simulink model "simulink_validacao"  (R2016a)
settings: Solver=VariableStepAuto  StartTime=0.0  StopTime=10.0  RelTol=1e-3
values from neighbouring files (symbols this model uses):
  f_mol_ar = [0.79 0.21 0.0 0 0 0 0 0]    [codigo_validacao.m]
  f_mol_gas = [0.76 0 0 0 0.11 0.13 0 0]    [codigo_validacao.m]
  m_c = 0.3    [codigo_validacao.m]
  m_f = 0.01    [codigo_validacao.m]
  N = 0.82    [codigo_validacao.m]
  Pc_i = 368000    [codigo_validacao.m]
  Ph_i = 105000    [codigo_validacao.m]
  Tc_i = 358.15    [codigo_validacao.m]
  Th_i = 584.817    [codigo_validacao.m]
(part 2 of 4)

== system simulink_validacao/Recuperdor de calor CWPS/Troca de Calor/Coef. Convectivo ==
  k_ar [W/m.K] : Inport
  k_gas [W/m.K] : Inport  Port=2
  nu_ar : Inport  Port=3
  nu_gas : Inport  Port=4
  dh_ar [m] : Inport  Port=5
  dh_gas [m] : Inport  Port=6
  Coeficiente Convectivo fluido frio : Fcn  Expr=u(1)*u(2)*(1/u(3))
  Coeficiente Convectivo fluido quente : Fcn  Expr=u(1)*u(2)*(1/u(3))
  Mux1 : Mux  Inputs=3
  Mux2 : Mux  Inputs=3
  coef-h_c [W/(m2.K)] : Outport
  coef-h_h [W/(m2.K)] : Outport  Port=2
  wires:
  nu_ar/1 -> Mux1/1
  nu_gas/1 -> Mux2/1
  k_ar [W/m.K]/1 -> Mux1/2
  k_gas [W/m.K]/1 -> Mux2/2
  Mux1/1 -> Coeficiente Convectivo fluido frio/1
  Coeficiente Convectivo fluido frio/1 -> coef-h_c [W/(m2.K)]/1
  dh_gas [m]/1 -> Mux2/3
  dh_ar [m]/1 -> Mux1/3
  Coeficiente Convectivo fluido quente/1 -> coef-h_h [W/(m2.K)]/1
  Mux2/1 -> Coeficiente Convectivo fluido quente/1

== system simulink_validacao/Recuperdor de calor CWPS/Troca de Calor/Coef. global ==
  coef-h_c [W/(m2.K)] : Inport
  coef-h_h [W/(m2.K)] : Inport  Port=2
  Calc. Coef. global : Fcn  Expr=(1/(u(1)*u(2)))+(1/(u(3)*u(4)))
  Mux1 : Mux
  cg [K/W] : Outport
  wires:
  coef-h_c [W/(m2.K)]/1 -> Mux1/1
  [Aht_h] -> Mux1/4
  coef-h_h [W/(m2.K)]/1 -> Mux1/3
  Calc. Coef. global/1 -> cg [K/W]/1
  Mux1/1 -> Calc. Coef. global/1
  [Aht_c] -> Mux1/2

== system simulink_validacao/Recuperdor de calor CWPS/Troca de Calor/Condutividade ==
  t_c_i [K] : Inport
  t_c_o [K] : Inport  Port=2
  t_h_i [K] : Inport  Port=3
  t_h_o [K] : Inport  Port=4
  Mux : Mux  Inputs=2
  Mux1 : Mux  Inputs=2
  T media fluido frio : Fcn  Expr=(u(1)+u(2))/2
  T media fluido quente : Fcn  Expr=(u(1)+u(2))/2
  cond_c_ch : MATLAB Function  TreatAsAtomicUnit=on
  cond_c_ch1 : MATLAB Function  TreatAsAtomicUnit=on
  k_c_ch [W/m.K] : Outport
  k_h_ch [W/m.K] : Outport  Port=2
  wires:
  Mux/1 -> T media fluido frio/1
  t_c_i [K]/1 -> Mux/1
  t_c_o [K]/1 -> Mux/2
  T media fluido frio/1 -> cond_c_ch/1(t)
  cond_c_ch/1(y) -> k_c_ch [W/m.K]/1
  Mux1/1 -> T media fluido quente/1
  t_h_i [K]/1 -> Mux1/1
  t_h_o [K]/1 -> Mux1/2
  T media fluido quente/1 -> cond_c_ch1/1(t)
  cond_c_ch1/1(y) -> k_h_ch [W/m.K]/1
  [f_mol_c] -> cond_c_ch/2(frac_mol)
  [f_mol_h] -> cond_c_ch1/2(frac_mol)

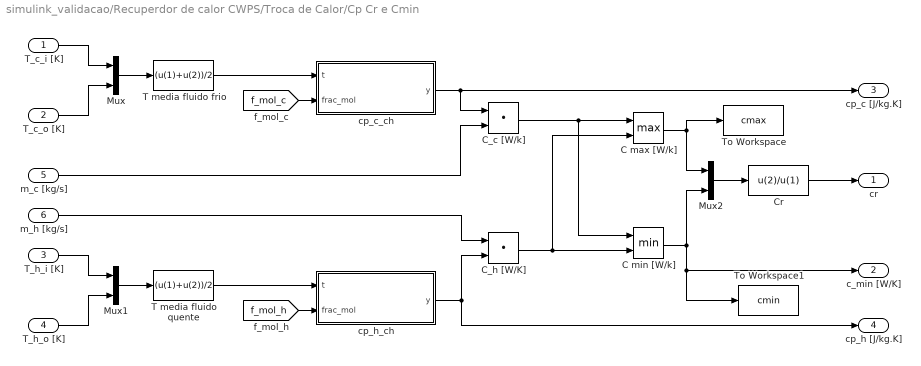
== system simulink_validacao/Recuperdor de calor CWPS/Troca de Calor/Cp Cr e Cmin ==
  T_c_i [K] : Inport
  T_c_o [K] : Inport  Port=2
  T_h_i [K] : Inport  Port=3
  T_h_o [K] : Inport  Port=4
  m_c [kg/s] : Inport  Port=5
  m_h [kg/s] : Inport  Port=6
  C max [W/k] : MinMax  Function=max  Inputs=2
  C min [W/k] : MinMax  Inputs=2
  C_c [W/k] : DotProduct  InputSameDT=on  OutDataTypeStr=Inherit: Inherit via internal rule
  C_h [W/K] : DotProduct  InputSameDT=on  OutDataTypeStr=Inherit: Inherit via internal rule
  Cr : Fcn  Expr=u(2)/u(1)
  Mux : Mux  Inputs=2
  Mux1 : Mux  Inputs=2
  Mux2 : Mux  Inputs=2
  T media fluido frio : Fcn  Expr=(u(1)+u(2))/2
  T media fluido quente : Fcn  Expr=(u(1)+u(2))/2
  To Workspace : ToWorkspace  VariableName=cmax  SampleTime=-1
      settings: Save2DSignal=2-D array (concatenate along first dimension)
  To Workspace1 : ToWorkspace  VariableName=cmin  SampleTime=-1
      settings: Save2DSignal=2-D array (concatenate along first dimension)
  cp_c_ch : MATLAB Function  TreatAsAtomicUnit=on
  cp_h_ch : MATLAB Function  TreatAsAtomicUnit=on
  cr : Outport
  c_min [W/K] : Outport  Port=2
  cp_c [J/kg.K] : Outport  Port=3
  cp_h [J/kg.K] : Outport  Port=4
  wires:
  Mux/1 -> T media fluido frio/1
  T_c_i [K]/1 -> Mux/1
  m_h [kg/s]/1 -> C_h [W/K]/1
  T media fluido quente/1 -> cp_h_ch/1(t)
  T_h_i [K]/1 -> Mux1/1
  C max [W/k]/1 -> Mux2/1, To Workspace/1
  cp_h_ch/1(y) -> C_h [W/K]/2, cp_h [J/kg.K]/1
  m_c [kg/s]/1 -> C_c [W/k]/2
  C_c [W/k]/1 -> C min [W/k]/1, C max [W/k]/1
  Cr/1 -> cr/1
  T_c_o [K]/1 -> Mux/2
  cp_c_ch/1(y) -> cp_c [J/kg.K]/1, C_c [W/k]/1
  T_h_o [K]/1 -> Mux1/2
  Mux2/1 -> Cr/1
  C_h [W/K]/1 -> C min [W/k]/2, C max [W/k]/2
  T media fluido frio/1 -> cp_c_ch/1(t)
  Mux1/1 -> T media fluido quente/1
  C min [W/k]/1 -> To Workspace1/1, c_min [W/K]/1, Mux2/2
  [f_mol_c] -> cp_c_ch/2(frac_mol)
  [f_mol_h] -> cp_h_ch/2(frac_mol)

== system simulink_validacao/Recuperdor de calor CWPS/Troca de Calor/Efetividade ==
  cr : Inport
  nut : Inport  Port=2
  Calc. Efetividade : Fcn  Expr=(1-exp(-u(2)*(1-u(1))))/(1-u(1)*exp(-u(2)*(1-u(1))))
  Mux1 : Mux  Inputs=2
  efetividade : ToWorkspace  VariableName=efetiv  SampleTime=-1
      settings: Save2DSignal=2-D array (concatenate along first dimension)
  epsilon : Outport
  wires:
  nut/1 -> Mux1/2
  cr/1 -> Mux1/1
  Calc. Efetividade/1 -> efetividade/1, epsilon/1
  Mux1/1 -> Calc. Efetividade/1

== system simulink_validacao/Recuperdor de calor CWPS/Troca de Calor/NUT ==
  c_min [W/K] : Inport
  cg [K/W] : Inport  Port=2
  Calc. NUT : Fcn  Expr=1/(u(1)*u(2))
  Mux1 : Mux  Inputs=2
  nut : Outport
  wires:
  cg [K/W]/1 -> Mux1/2
  c_min [W/K]/1 -> Mux1/1
  Calc. NUT/1 -> nut/1
  Mux1/1 -> Calc. NUT/1

== system simulink_validacao/Recuperdor de calor CWPS/Troca de Calor/Nusselt ==
  pr_ar : Inport
  pr_gas : Inport  Port=2
  re_ar : Inport  Port=3
  re_gas : Inport  Port=4
  Calc. Nusselt ar : Fcn  Expr=0.0031*(u(1)^1.18)*(u(2)^0.4)*((2*u(3)/u(4))^0.19)
  Calc. Nusselt gas : Fcn  Expr=0.0031*(u(1)^1.18)*(u(2)^0.4)*((2*u(3)/u(4))^0.19)
  Mux1 : Mux
  Mux2 : Mux
  nu_ar : Outport
  nu_gas : Outport  Port=2
  wires:
  pr_ar/1 -> Mux1/2
  Mux2/1 -> Calc. Nusselt gas/1
  Calc. Nusselt gas/1 -> nu_gas/1
  re_ar/1 -> Mux1/1
  re_gas/1 -> Mux2/1
  [W_c] -> Mux1/4
  [h] -> Mux2/3, Mux1/3
  Calc. Nusselt ar/1 -> nu_ar/1
  Mux1/1 -> Calc. Nusselt ar/1
  [W_h] -> Mux2/4
  pr_gas/1 -> Mux2/2

== system simulink_validacao/Recuperdor de calor CWPS/Troca de Calor/Prandlt ==
  cp_ar [J/kg.K] : Inport
  cp_gas [J/kg.K] : Inport  Port=2
  mu_ar [kg/m.s] : Inport  Port=3
  mu_gas [kg/m.s] : Inport  Port=4
  k_ar_ch [W/m.K] : Inport  Port=5
  k_gas_ch  [W/m.K] : Inport  Port=6
  Mux : Mux  Inputs=3
  Mux1 : Mux  Inputs=3
  Prandlt fluido frio : Fcn  Expr=(u(1)*u(2))/(u(3))
  Prandlt fluido quente : Fcn  Expr=(u(1)*u(2))/(u(3))
  pr_c : Outport
  pr_h : Outport  Port=2
  wires:
  Mux1/1 -> Prandlt fluido quente/1
  Prandlt fluido quente/1 -> pr_h/1
  k_gas_ch  [W/m.K]/1 -> Mux1/3
  cp_gas [J/kg.K]/1 -> Mux1/1
  mu_ar [kg/m.s]/1 -> Mux/2
  Mux/1 -> Prandlt fluido frio/1
  Prandlt fluido frio/1 -> pr_c/1
  mu_gas [kg/m.s]/1 -> Mux1/2
  cp_ar [J/kg.K]/1 -> Mux/1
  k_ar_ch [W/m.K]/1 -> Mux/3

== system simulink_validacao/Recuperdor de calor CWPS/Troca de Calor/Taxa Calor ==
  c_min [W/K] : Inport
  epsilon : Inport  Port=2
  T_c_i [K] : Inport  Port=3
  T_h_i [K] : Inport  Port=4
  Mux1 : Mux
  Taxa Transf calor real : Fcn  Expr=u(1)*u(2)*(u(3)-u(4))
  Taxa de Transferência : ToWorkspace  VariableName=q_dot  SampleTime=-1
      settings: Save2DSignal=2-D array (concatenate along first dimension)
  Q [W] : Outport
  wires:
  Mux1/1 -> Taxa Transf calor real/1
  Taxa Transf calor real/1 -> Taxa de Transferência/1, Q [W]/1
  T_c_i [K]/1 -> Mux1/4
  T_h_i [K]/1 -> Mux1/3
  c_min [W/K]/1 -> Mux1/2
  epsilon/1 -> Mux1/1

== system simulink_validacao/Recuperdor de calor CWPS/Troca de Calor/Transf calor ==
  Q [W] : Inport
  T_h_i [K] : Inport  Port=2
  T_c_i [K] : Inport  Port=3
  cp_c [J/kg.K] : Inport  Port=4
  cp_h [J/kg.K] : Inport  Port=5
  m_c [kg/s] : Inport  Port=6
  "m_h [kg/s] " : Inport  Port=7
  Mux1 : Mux
  Mux2 : Mux
  Taxa de transferência de calor fluido frio : Fcn  Expr=(u(4)/(u(1)*u(2)))+u(3)
  "Taxa de transferência de calor fluido quente " : Fcn  Expr=u(3)-(u(4)/(u(1)*u(2)))
  T_c_o [K] : Outport
  T_h_o [K] : Outport  Port=2
  wires:
  Mux1/1 -> Taxa de transferência de calor fluido frio/1
  Taxa de transferência de calor fluido frio/1 -> T_c_o [K]/1
  Mux2/1 -> "Taxa de transferência de calor fluido quente "/1
  "Taxa de transferência de calor fluido quente "/1 -> T_h_o [K]/1
  m_c [kg/s]/1 -> Mux1/1
  cp_c [J/kg.K]/1 -> Mux1/2
  T_c_i [K]/1 -> Mux1/3
  Q [W]/1 -> Mux2/4, Mux1/4
  cp_h [J/kg.K]/1 -> Mux2/2
  T_h_i [K]/1 -> Mux2/3
  "m_h [kg/s] "/1 -> Mux2/1

== matlab function simulink_validacao/Recuperdor de calor CWPS/Densidade Fluido Frio/densidade_c_o ==
  data: t input; y output; p input; frac_mol input
function y = rho(t,p,frac_mol)
%#codegen
%
%------------------- FUNÇÃO DENSIDADE DOS GASES -------------------------
%
%   -Autor: Janderson Honório Mazzine Afonso
%   -Email: janderson.mazzine2015@engenharia.ufjf.br
%   -Ano: 2020
%   -Referência: IUPAC. Periodic Table of Elements. Disponivel em
%   <https://iupac.org/what-we-do/periodic-table-of-elements/> Acesso em
%   01 set. 2020.
%   -Citar como: AFONSO. Janderson H. M. Densidade dos Gases de Combustão
%                Aplicados em Turbinas a Gás. UFJF, 2020.
%   -Versão: 01.09.2020
%
%----------------------- DESCRIÇÃO DA FUNÇÃO ------------------------------
%
%   A presente função retorna a densidade, em [kg/m^3] de um gás puro ou 
%   mistura de gases ideais segundo a equação de Clapeyron, considerando as
%   massas molares dos atomos na tabela da IUPAC
%
%--------------------------- INSTRUÇÕES -----------------------------------
%
%              [rho] = densi_gas( t, p, frac_mol)
%
%   A temperatura de entrada deve ser dada em Kelvin [K], a pressão em mega
%   Pascal [Pa]. As frações molares devem ser dada em um vetor com o  
%   seguinte formato:
%
%                 (%N2 %O2 %Ar %Ne %H2O %CO2 %CO %SO2)
%
%   Caso alguma das espécies não faça parte da mistura deve ser atribuido o
%   valor 0 (zero) a sua posição no vetor. A soma das frações de cada espé-
%   cie deve ser sempre igual a 1.
%
%------------------------ MENSAGEM DE ERRO -------------------------------- 
%
%   Uma mensagem de erro será exibida caso a soma das concentrações dos 
%   componentes do gás em estudo seja diferente de 1.
%
%---------------------------- EXEMPLOS ------------------------------------
%
%   1)Definir a densidade do ar atmosférico considerando uma composição de 
%   Oxigênio (21%) e Nitrogênio (79%) apenas, a 100ºC e 2 atm.
%
%   t = 373.15;
%   p = 0.202650;
%   frac_mol = [0.79 0.21 0 0 0 0 0 0];
%   [rho] = densi_gas( t, p, frac_mol);
%
%   ANS: 1.88444931513629e+000
%   
%--------------------------------------------------------------------------

if  sum(frac_mol) ~= 1 %checa composição informada
    error('A soma das frações de composição é diferente de 1')
end

mm_el = [28.014 31.998 39.95 20.180 33.006 44.009 28.01 64.058]; %massa molar dos gases puros segundo IUPAC 2020, [g/mol]

rho = 0; 
R=8.314462; %Constante dos gases, em [m^3 Pa kg^-1 mol^-1]
    for j = 1:8, %percorre espécies
        if frac_mol(j) > 0  %evita o cálculo das especies com concentração nula
            rho=rho+(((mm_el(j)*10^(-3))*frac_mol(j)*(p))/(R*t)); 
        end
    end
    
    y = rho;

== matlab function simulink_validacao/Recuperdor de calor CWPS/Densidade Fluido Frio/densidade_c_i ==
  data: t input; y output; p input; frac_mol input
function y = rho(t,p,frac_mol)
%#codegen
%
%------------------- FUNÇÃO DENSIDADE DOS GASES -------------------------
%
%   -Autor: Janderson Honório Mazzine Afonso
%   -Email: janderson.mazzine2015@engenharia.ufjf.br
%   -Ano: 2020
%   -Referência: IUPAC. Periodic Table of Elements. Disponivel em
%   <https://iupac.org/what-we-do/periodic-table-of-elements/> Acesso em
%   01 set. 2020.
%   -Citar como: AFONSO. Janderson H. M. Densidade dos Gases de Combustão
%                Aplicados em Turbinas a Gás. UFJF, 2020.
%   -Versão: 01.09.2020
%
%----------------------- DESCRIÇÃO DA FUNÇÃO ------------------------------
%
%   A presente função retorna a densidade, em [kg/m^3] de um gás puro ou 
%   mistura de gases ideais segundo a equação de Clapeyron, considerando as
%   massas molares dos atomos na tabela da IUPAC
%
%--------------------------- INSTRUÇÕES -----------------------------------
%
%              [rho] = densi_gas( t, p, frac_mol)
%
%   A temperatura de entrada deve ser dada em Kelvin [K], a pressão em mega
%   Pascal [Pa]. As frações molares devem ser dada em um vetor com o  
%   seguinte formato:
%
%                 (%N2 %O2 %Ar %Ne %H2O %CO2 %CO %SO2)
%
%   Caso alguma das espécies não faça parte da mistura deve ser atribuido o
%   valor 0 (zero) a sua posição no vetor. A soma das frações de cada espé-
%   cie deve ser sempre igual a 1.
%
%------------------------ MENSAGEM DE ERRO -------------------------------- 
%
%   Uma mensagem de erro será exibida caso a soma das concentrações dos 
%   componentes do gás em estudo seja diferente de 1.
%
%---------------------------- EXEMPLOS ------------------------------------
%
%   1)Definir a densidade do ar atmosférico considerando uma composição de 
%   Oxigênio (21%) e Nitrogênio (79%) apenas, a 100ºC e 2 atm.
%
%   t = 373.15;
%   p = 0.202650;
%   frac_mol = [0.79 0.21 0 0 0 0 0 0];
%   [rho] = densi_gas( t, p, frac_mol);
%
%   ANS: 1.88444931513629e+000
%   
%--------------------------------------------------------------------------

if  sum(frac_mol) ~= 1 %checa composição informada
    error('A soma das frações de composição é diferente de 1')
end

mm_el = [28.014 31.998 39.95 20.180 33.006 44.009 28.01 64.058]; %massa molar dos gases puros segundo IUPAC 2020, [g/mol]

rho = 0; 
R=8.314462; %Constante dos gases, em [m^3 Pa kg^-1 mol^-1]
    for j = 1:8, %percorre espécies
        if frac_mol(j) > 0  %evita o cálculo das especies com concentração nula
            rho=rho+(((mm_el(j)*10^(-3))*frac_mol(j)*(p))/(R*t)); 
        end
    end
    
    y = rho;

== matlab function simulink_validacao/Recuperdor de calor CWPS/Densidade Fluido Quente/densidade_h_ch ==
  data: t input; y output; p input; frac_mol input
function y = rho(t,p,frac_mol)
%#codegen
%
%------------------- FUNÇÃO DENSIDADE DOS GASES -------------------------
%
%   -Autor: Janderson Honório Mazzine Afonso
%   -Email: janderson.mazzine2015@engenharia.ufjf.br
%   -Ano: 2020
%   -Referência: IUPAC. Periodic Table of Elements. Disponivel em
%   <https://iupac.org/what-we-do/periodic-table-of-elements/> Acesso em
%   01 set. 2020.
%   -Citar como: AFONSO. Janderson H. M. Densidade dos Gases de Combustão
%                Aplicados em Turbinas a Gás. UFJF, 2020.
%   -Versão: 01.09.2020
%
%----------------------- DESCRIÇÃO DA FUNÇÃO ------------------------------
%
%   A presente função retorna a densidade, em [kg/m^3] de um gás puro ou 
%   mistura de gases ideais segundo a equação de Clapeyron, considerando as
%   massas molares dos atomos na tabela da IUPAC
%
%--------------------------- INSTRUÇÕES -----------------------------------
%
%              [rho] = densi_gas( t, p, frac_mol)
%
%   A temperatura de entrada deve ser dada em Kelvin [K], a pressão em mega
%   Pascal [Pa]. As frações molares devem ser dada em um vetor com o  
%   seguinte formato:
%
%                 (%N2 %O2 %Ar %Ne %H2O %CO2 %CO %SO2)
%
%   Caso alguma das espécies não faça parte da mistura deve ser atribuido o
%   valor 0 (zero) a sua posição no vetor. A soma das frações de cada espé-
%   cie deve ser sempre igual a 1.
%
%------------------------ MENSAGEM DE ERRO -------------------------------- 
%
%   Uma mensagem de erro será exibida caso a soma das concentrações dos 
%   componentes do gás em estudo seja diferente de 1.
%
%---------------------------- EXEMPLOS ------------------------------------
%
%   1)Definir a densidade do ar atmosférico considerando uma composição de 
%   Oxigênio (21%) e Nitrogênio (79%) apenas, a 100ºC e 2 atm.
%
%   t = 373.15;
%   p = 0.202650;
%   frac_mol = [0.79 0.21 0 0 0 0 0 0];
%   [rho] = densi_gas( t, p, frac_mol);
%
%   ANS: 1.88444931513629e+000
%   
%--------------------------------------------------------------------------

if  sum(frac_mol) ~= 1 %checa composição informada
    error('A soma das frações de composição é diferente de 1')
end

mm_el = [28.014 31.998 39.95 20.180 33.006 44.009 28.01 64.058]; %massa molar dos gases puros segundo IUPAC 2020, [g/mol]

rho = 0; 
R=8.314462; %Constante dos gases, em [m^3 Pa kg^-1 mol^-1]
    for j = 1:8, %percorre espécies
        if frac_mol(j) > 0  %evita o cálculo das especies com concentração nula
            rho=rho+(((mm_el(j)*10^(-3))*frac_mol(j)*(p))/(R*t)); 
        end
    end
    
    y = rho;

== matlab function simulink_validacao/Recuperdor de calor CWPS/Viscosidade Fluido Frio /visc_c_c ==
  data: t input; y output; frac_mol input
function y = mu(t, frac_mol)
%#codegen
%------------------- FUNÇÃO VISCOSIDADE DOS GASES -------------------------
%
%   -Autor: Janderson Honório Mazzine Afonso
%   -Email: janderson.mazzine2015@engenharia.ufjf.br
%   -Ano: 2020
%
%   -Referências: 
%   [1]MATOS, M. A. A. Propriedades termofísicas de algunsgases, sólidos e  
%   da água. Aveiro: Editora da Universidade de Aveiro, 1998.
%   [2]BIRD R. B., WARREN E. S., and EDWIN N. L. Transport Phenomena. 2nd 
%   ed. New York: Jonh Wiley & Sons, 2002.
%   [3]IUPAC. Periodic Table of Elements. Disponivel em
%   <https://iupac.org/what-we-do/periodic-table-of-elements/> Acesso em
%   01 set. 2020.
%
%   -Citar como: AFONSO. Janderson H. M. Vicosidade dos Gases de Combustão
%                Aplicados em Turbinas a Gás. UFJF, 2020.
%   -Versão: 01.09.2020
%
%----------------------- DESCRIÇÃO DA FUNÇÃO ------------------------------
%
%   A presente função retorna a viscosidade dinâmica, em [kg/m.s] de um gás 
%   puro segundo a expressão e coeicientes de regressão apresentados por  
%   Matos [1], e da mistura considerando também a correlação semiempírica 
%   desenvolvida por Wilke e apresentada no livro de Bird [2], considerando 
%   as massas molares dos atomos na tabela da IUPAC [3].
%
%--------------------------- INSTRUÇÕES -----------------------------------
%
%                   [mu] = visc_gas( t, frac_mol)
%
%   A temperatura de entrada deve ser dada em Kelvin [K] e as frações 
%   molares devem ser dada em um vetor com o seguinte formato:
%   
%                 (%N2 %O2 %Ar %Ne %H2O %CO2 %CO %SO2)
%
%   Caso alguma das espécies não faça parte da mistura deve ser atribuido o
%   valor 0 (zero) a sua posição no vetor. A soma das frações de cada espé-
%   cie deve ser sempre igual a 1.
%   
%   Porém, o presente modelo não contempla o gas neônio. Caso seja
%   necessário, deve-se implementar seus coeficientes na matriz.
%
%-------------------- MENSAGEM DE ERRO E AVISOS --------------------------- 
%
%   Uma mensagem de erro será exibida caso a soma das concentrações dos 
%   componentes do gás em estudo seja diferente de 1, ou caso tente-se 
%   computar um gás que possua Neônio em sua composição, o qual não é 
%   contemplado no presente modelo.
%   
%   Um aviso será exibido caso a temperatura desejada da mistura esteja
%   fora do intervalo de temperatura de algum dos gases puros que a compõe,
%   conforme a tabela abaixo:
%
%              Gas	|	T_min (K)	|	T_max (K)
%               ---------------------------------
%               N2 		  250 			  1500
%               O2		  250 			  1500
%               Ar		  250			  1300
%               Ne		  NaN			  NaN
%               H2O 	  400 			  1500
%               CO2 	  250 			  1500 
%               CO		  250 			  1500
%               SO2 	  170 			  1700
%
%---------------------------- EXEMPLOS ------------------------------------
%
%   1)Definir a viscosidade do ar atmosférico considerando uma composição 
%   de Oxigênio (21%) e Nitrogênio (79%) apenas, a 100ºC.
%
%   t = 373.15;
%   f_mol = [0.79 0.21 0 0 0 0 0 0];
%
%   ANS: 21.8025339818354e-006
%   
%--------------------------------------------------------------------------


if  sum(frac_mol) ~= 1 %checa composição informada
    error('A soma das frações de composição é diferente de 1');
elseif frac_mol(4) ~= 0
    error('Erro: Gás Neonio não contemplado no modelo');
end


mm_el = [28.014 31.998 39.95 20.180 33.006 44.009 28.01 64.058]; %massa molar dos gases puros segundo IUPAC 2020, [g/mol]

mu = 0;
cont = 0;
vis = zeros(1, 8);
fm = zeros(1, 8);
mm = zeros(1, 8);
psi_ab = zeros(1, 8);

coef = [0.31619*10^(-5)		0.56192*10^(-7) 	-0.24148*10^(-10)  	0.61370*10^(-14) 	250 	1500;
        0.26918*10^(-5)		0.68519*10^(-7)  	-0.29857*10^(-10) 	0.75600*10^(-14) 	250 	1500;
        0.50458*10^(-5)		0.63459*10^(-7)  	-0.17506*10^(-10) 	0.37009*10^(-14) 	250     1300;
        0                   0                   0                   0                   0       0;
        -0.41991*10^(-5) 	0.45336E-07    		-0.50749*10^(-11) 	0.15526*10^(-14) 	400 	1500;
        -0.16636*10^(-5)	0.63064*10^(-7)  	-0.26223*10^(-10) 	0.58813*10^(-14) 	250 	1500; 
        0.30012*10^(-5)		0.56504*10^(-7)  	-0.23998*10^(-10) 	0.62734*10^(-14) 	250 	1500; 
        0-.37930*10^(-5)	0.46450*10^(-7) 	-0.72760*10^(-11) 	0                   170 	1700];

    for i = 1:8, %percorre espécies
        if frac_mol(i) ~= 0  %evita o cálculo das especies com concentração nula
            cont=cont+1;
            fm(cont)= frac_mol(i);
            mm(cont)= mm_el(i);
            vis(cont)=coef(i,1)+coef(i,2)*t+coef(i,3)*t^2+coef(i,4)*t^3;
            if t<coef(i,5)
                error('A temperatura está abaixo do limite de aplicabilidade do modelo para o gas abaixo:')
            elseif t>coef(i,6)
                error('A temperatura está acima do limite de aplicabilidade do modelo para os gas abaixo:')
            end
        end
    end
    
    for a = 1:cont, %calculo psi
        for b = 1:cont,
            psi_ab(a)=psi_ab(a)+fm(b)*((1/sqrt(8))*(1+mm(a)/mm(b))^(-0.5)*(1+(vis(a)/vis(b))^(0.5)*(mm(b)/mm(a))^(0.25))^2);
        end
        mu=mu+((fm(a)*vis(a))/psi_ab(a));
    end
    y = mu;

== matlab function simulink_validacao/Recuperdor de calor CWPS/Viscosidade Fluido Frio /visc_c_o ==
  data: t input; y output; frac_mol input
function y = mu(t, frac_mol)
%#codegen
%------------------- FUNÇÃO VISCOSIDADE DOS GASES -------------------------
%
%   -Autor: Janderson Honório Mazzine Afonso
%   -Email: janderson.mazzine2015@engenharia.ufjf.br
%   -Ano: 2020
%
%   -Referências: 
%   [1]MATOS, M. A. A. Propriedades termofísicas de algunsgases, sólidos e  
%   da água. Aveiro: Editora da Universidade de Aveiro, 1998.
%   [2]BIRD R. B., WARREN E. S., and EDWIN N. L. Transport Phenomena. 2nd 
%   ed. New York: Jonh Wiley & Sons, 2002.
%   [3]IUPAC. Periodic Table of Elements. Disponivel em
%   <https://iupac.org/what-we-do/periodic-table-of-elements/> Acesso em
%   01 set. 2020.
%
%   -Citar como: AFONSO. Janderson H. M. Vicosidade dos Gases de Combustão
%                Aplicados em Turbinas a Gás. UFJF, 2020.
%   -Versão: 01.09.2020
%
%----------------------- DESCRIÇÃO DA FUNÇÃO ------------------------------
%
%   A presente função retorna a viscosidade dinâmica, em [kg/m.s] de um gás 
%   puro segundo a expressão e coeicientes de regressão apresentados por  
%   Matos [1], e da mistura considerando também a correlação semiempírica 
%   desenvolvida por Wilke e apresentada no livro de Bird [2], considerando 
%   as massas molares dos atomos na tabela da IUPAC [3].
%
%--------------------------- INSTRUÇÕES -----------------------------------
%
%                   [mu] = visc_gas( t, frac_mol)
%
%   A temperatura de entrada deve ser dada em Kelvin [K] e as frações 
%   molares devem ser dada em um vetor com o seguinte formato:
%   
%                 (%N2 %O2 %Ar %Ne %H2O %CO2 %CO %SO2)
%
%   Caso alguma das espécies não faça parte da mistura deve ser atribuido o
%   valor 0 (zero) a sua posição no vetor. A soma das frações de cada espé-
%   cie deve ser sempre igual a 1.
%   
%   Porém, o presente modelo não contempla o gas neônio. Caso seja
%   necessário, deve-se implementar seus coeficientes na matriz.
%
%-------------------- MENSAGEM DE ERRO E AVISOS --------------------------- 
%
%   Uma mensagem de erro será exibida caso a soma das concentrações dos 
%   componentes do gás em estudo seja diferente de 1, ou caso tente-se 
%   computar um gás que possua Neônio em sua composição, o qual não é 
%   contemplado no presente modelo.
%   
%   Um aviso será exibido caso a temperatura desejada da mistura esteja
%   fora do intervalo de temperatura de algum dos gases puros que a compõe,
%   conforme a tabela abaixo:
%
%              Gas	|	T_min (K)	|	T_max (K)
%               ---------------------------------
%               N2 		  250 			  1500
%               O2		  250 			  1500
%               Ar		  250			  1300
%               Ne		  NaN			  NaN
%               H2O 	  400 			  1500
%               CO2 	  250 			  1500 
%               CO		  250 			  1500
%               SO2 	  170 			  1700
%
%---------------------------- EXEMPLOS ------------------------------------
%
%   1)Definir a viscosidade do ar atmosférico considerando uma composição 
%   de Oxigênio (21%) e Nitrogênio (79%) apenas, a 100ºC.
%
%   t = 373.15;
%   f_mol = [0.79 0.21 0 0 0 0 0 0];
%
%   ANS: 21.8025339818354e-006
%   
%--------------------------------------------------------------------------


if  sum(frac_mol) ~= 1 %checa composição informada
    error('A soma das frações de composição é diferente de 1');
elseif frac_mol(4) ~= 0
    error('Erro: Gás Neonio não contemplado no modelo');
end


mm_el = [28.014 31.998 39.95 20.180 33.006 44.009 28.01 64.058]; %massa molar dos gases puros segundo IUPAC 2020, [g/mol]

mu = 0;
cont = 0;
vis = zeros(1, 8);
fm = zeros(1, 8);
mm = zeros(1, 8);
psi_ab = zeros(1, 8);

coef = [0.31619*10^(-5)		0.56192*10^(-7) 	-0.24148*10^(-10)  	0.61370*10^(-14) 	250 	1500;
        0.26918*10^(-5)		0.68519*10^(-7)  	-0.29857*10^(-10) 	0.75600*10^(-14) 	250 	1500;
        0.50458*10^(-5)		0.63459*10^(-7)  	-0.17506*10^(-10) 	0.37009*10^(-14) 	250     1300;
        0                   0                   0                   0                   0       0;
        -0.41991*10^(-5) 	0.45336E-07    		-0.50749*10^(-11) 	0.15526*10^(-14) 	400 	1500;
        -0.16636*10^(-5)	0.63064*10^(-7)  	-0.26223*10^(-10) 	0.58813*10^(-14) 	250 	1500; 
        0.30012*10^(-5)		0.56504*10^(-7)  	-0.23998*10^(-10) 	0.62734*10^(-14) 	250 	1500; 
        0-.37930*10^(-5)	0.46450*10^(-7) 	-0.72760*10^(-11) 	0                   170 	1700];

    for i = 1:8, %percorre espécies
        if frac_mol(i) ~= 0  %evita o cálculo das especies com concentração nula
            cont=cont+1;
            fm(cont)= frac_mol(i);
            mm(cont)= mm_el(i);
            vis(cont)=coef(i,1)+coef(i,2)*t+coef(i,3)*t^2+coef(i,4)*t^3;
            if t<coef(i,5)
                error('A temperatura está abaixo do limite de aplicabilidade do modelo para o gas abaixo:')
            elseif t>coef(i,6)
                error('A temperatura está acima do limite de aplicabilidade do modelo para os gas abaixo:')
            end
        end
    end
    
    for a = 1:cont, %calculo psi
        for b = 1:cont,
            psi_ab(a)=psi_ab(a)+fm(b)*((1/sqrt(8))*(1+mm(a)/mm(b))^(-0.5)*(1+(vis(a)/vis(b))^(0.5)*(mm(b)/mm(a))^(0.25))^2);
        end
        mu=mu+((fm(a)*vis(a))/psi_ab(a));
    end
    y = mu;

== matlab function simulink_validacao/Recuperdor de calor CWPS/Viscosidade Fluido Frio /visc_c_ch ==
  data: t input; y output; frac_mol input
function y = mu(t, frac_mol)
%#codegen
%------------------- FUNÇÃO VISCOSIDADE DOS GASES -------------------------
%
%   -Autor: Janderson Honório Mazzine Afonso
%   -Email: janderson.mazzine2015@engenharia.ufjf.br
%   -Ano: 2020
%
%   -Referências: 
%   [1]MATOS, M. A. A. Propriedades termofísicas de algunsgases, sólidos e  
%   da água. Aveiro: Editora da Universidade de Aveiro, 1998.
%   [2]BIRD R. B., WARREN E. S., and EDWIN N. L. Transport Phenomena. 2nd 
%   ed. New York: Jonh Wiley & Sons, 2002.
%   [3]IUPAC. Periodic Table of Elements. Disponivel em
%   <https://iupac.org/what-we-do/periodic-table-of-elements/> Acesso em
%   01 set. 2020.
%
%   -Citar como: AFONSO. Janderson H. M. Vicosidade dos Gases de Combustão
%                Aplicados em Turbinas a Gás. UFJF, 2020.
%   -Versão: 01.09.2020
%
%----------------------- DESCRIÇÃO DA FUNÇÃO ------------------------------
%
%   A presente função retorna a viscosidade dinâmica, em [kg/m.s] de um gás 
%   puro segundo a expressão e coeicientes de regressão apresentados por  
%   Matos [1], e da mistura considerando também a correlação semiempírica 
%   desenvolvida por Wilke e apresentada no livro de Bird [2], considerando 
%   as massas molares dos atomos na tabela da IUPAC [3].
%
%--------------------------- INSTRUÇÕES -----------------------------------
%
%                   [mu] = visc_gas( t, frac_mol)
%
%   A temperatura de entrada deve ser dada em Kelvin [K] e as frações 
%   molares devem ser dada em um vetor com o seguinte formato:
%   
%                 (%N2 %O2 %Ar %Ne %H2O %CO2 %CO %SO2)
%
%   Caso alguma das espécies não faça parte da mistura deve ser atribuido o
%   valor 0 (zero) a sua posição no vetor. A soma das frações de cada espé-
%   cie deve ser sempre igual a 1.
%   
%   Porém, o presente modelo não contempla o gas neônio. Caso seja
%   necessário, deve-se implementar seus coeficientes na matriz.
%
%-------------------- MENSAGEM DE ERRO E AVISOS --------------------------- 
%
%   Uma mensagem de erro será exibida caso a soma das concentrações dos 
%   componentes do gás em estudo seja diferente de 1, ou caso tente-se 
%   computar um gás que possua Neônio em sua composição, o qual não é 
%   contemplado no presente modelo.
%   
%   Um aviso será exibido caso a temperatura desejada da mistura esteja
%   fora do intervalo de temperatura de algum dos gases puros que a compõe,
%   conforme a tabela abaixo:
%
%              Gas	|	T_min (K)	|	T_max (K)
%               ---------------------------------
%               N2 		  250 			  1500
%               O2		  250 			  1500
%               Ar		  250			  1300
%               Ne		  NaN			  NaN
%               H2O 	  400 			  1500
%               CO2 	  250 			  1500 
%               CO		  250 			  1500
%               SO2 	  170 			  1700
%
%---------------------------- EXEMPLOS ------------------------------------
%
%   1)Definir a viscosidade do ar atmosférico considerando uma composição 
%   de Oxigênio (21%) e Nitrogênio (79%) apenas, a 100ºC.
%
%   t = 373.15;
%   f_mol = [0.79 0.21 0 0 0 0 0 0];
%
%   ANS: 21.8025339818354e-006
%   
%--------------------------------------------------------------------------


if  sum(frac_mol) ~= 1 %checa composição informada
    error('A soma das frações de composição é diferente de 1');
elseif frac_mol(4) ~= 0
    error('Erro: Gás Neonio não contemplado no modelo');
end


mm_el = [28.014 31.998 39.95 20.180 33.006 44.009 28.01 64.058]; %massa molar dos gases puros segundo IUPAC 2020, [g/mol]

mu = 0;
cont = 0;
vis = zeros(1, 8);
fm = zeros(1, 8);
mm = zeros(1, 8);
psi_ab = zeros(1, 8);

coef = [0.31619*10^(-5)		0.56192*10^(-7) 	-0.24148*10^(-10)  	0.61370*10^(-14) 	250 	1500;
        0.26918*10^(-5)		0.68519*10^(-7)  	-0.29857*10^(-10) 	0.75600*10^(-14) 	250 	1500;
        0.50458*10^(-5)		0.63459*10^(-7)  	-0.17506*10^(-10) 	0.37009*10^(-14) 	250     1300;
        0                   0                   0                   0                   0       0;
        -0.41991*10^(-5) 	0.45336E-07    		-0.50749*10^(-11) 	0.15526*10^(-14) 	400 	1500;
        -0.16636*10^(-5)	0.63064*10^(-7)  	-0.26223*10^(-10) 	0.58813*10^(-14) 	250 	1500; 
        0.30012*10^(-5)		0.56504*10^(-7)  	-0.23998*10^(-10) 	0.62734*10^(-14) 	250 	1500; 
        0-.37930*10^(-5)	0.46450*10^(-7) 	-0.72760*10^(-11) 	0                   170 	1700];

    for i = 1:8, %percorre espécies
        if frac_mol(i) ~= 0  %evita o cálculo das especies com concentração nula
            cont=cont+1;
            fm(cont)= frac_mol(i);
            mm(cont)= mm_el(i);
            vis(cont)=coef(i,1)+coef(i,2)*t+coef(i,3)*t^2+coef(i,4)*t^3;
            if t<coef(i,5)
                error('A temperatura está abaixo do limite de aplicabilidade do modelo para o gas abaixo:')
            elseif t>coef(i,6)
                error('A temperatura está acima do limite de aplicabilidade do modelo para os gas abaixo:')
            end
        end
    end
    
    for a = 1:cont, %calculo psi
        for b = 1:cont,
            psi_ab(a)=psi_ab(a)+fm(b)*((1/sqrt(8))*(1+mm(a)/mm(b))^(-0.5)*(1+(vis(a)/vis(b))^(0.5)*(mm(b)/mm(a))^(0.25))^2);
        end
        mu=mu+((fm(a)*vis(a))/psi_ab(a));
    end
    y = mu;

== matlab function simulink_validacao/Recuperdor de calor CWPS/Viscosidade Fluido Quente/visc_h_ch ==
  data: t input; y output; frac_mol input
function y = mu(t, frac_mol)
%#codegen
%------------------- FUNÇÃO VISCOSIDADE DOS GASES -------------------------
%
%   -Autor: Janderson Honório Mazzine Afonso
%   -Email: janderson.mazzine2015@engenharia.ufjf.br
%   -Ano: 2020
%
%   -Referências: 
%   [1]MATOS, M. A. A. Propriedades termofísicas de algunsgases, sólidos e  
%   da água. Aveiro: Editora da Universidade de Aveiro, 1998.
%   [2]BIRD R. B., WARREN E. S., and EDWIN N. L. Transport Phenomena. 2nd 
%   ed. New York: Jonh Wiley & Sons, 2002.
%   [3]IUPAC. Periodic Table of Elements. Disponivel em
%   <https://iupac.org/what-we-do/periodic-table-of-elements/> Acesso em
%   01 set. 2020.
%
%   -Citar como: AFONSO. Janderson H. M. Vicosidade dos Gases de Combustão
%                Aplicados em Turbinas a Gás. UFJF, 2020.
%   -Versão: 01.09.2020
%
%----------------------- DESCRIÇÃO DA FUNÇÃO ------------------------------
%
%   A presente função retorna a viscosidade dinâmica, em [kg/m.s] de um gás 
%   puro segundo a expressão e coeicientes de regressão apresentados por  
%   Matos [1], e da mistura considerando também a correlação semiempírica 
%   desenvolvida por Wilke e apresentada no livro de Bird [2], considerando 
%   as massas molares dos atomos na tabela da IUPAC [3].
%
%--------------------------- INSTRUÇÕES -----------------------------------
%
%                   [mu] = visc_gas( t, frac_mol)
%
%   A temperatura de entrada deve ser dada em Kelvin [K] e as frações 
%   molares devem ser dada em um vetor com o seguinte formato:
%   
%                 (%N2 %O2 %Ar %Ne %H2O %CO2 %CO %SO2)
%
%   Caso alguma das espécies não faça parte da mistura deve ser atribuido o
%   valor 0 (zero) a sua posição no vetor. A soma das frações de cada espé-
%   cie deve ser sempre igual a 1.
%   
%   Porém, o presente modelo não contempla o gas neônio. Caso seja
%   necessário, deve-se implementar seus coeficientes na matriz.
%
%-------------------- MENSAGEM DE ERRO E AVISOS --------------------------- 
%
%   Uma mensagem de erro será exibida caso a soma das concentrações dos 
%   componentes do gás em estudo seja diferente de 1, ou caso tente-se 
%   computar um gás que possua Neônio em sua composição, o qual não é 
%   contemplado no presente modelo.
%   
%   Um aviso será exibido caso a temperatura desejada da mistura esteja
%   fora do intervalo de temperatura de algum dos gases puros que a compõe,
%   conforme a tabela abaixo:
%
%              Gas	|	T_min (K)	|	T_max (K)
%               ---------------------------------
%               N2 		  250 			  1500
%               O2		  250 			  1500
%               Ar		  250			  1300
%               Ne		  NaN			  NaN
%               H2O 	  400 			  1500
%               CO2 	  250 			  1500 
%               CO		  250 			  1500
%               SO2 	  170 			  1700
%
%---------------------------- EXEMPLOS ------------------------------------
%
%   1)Definir a viscosidade do ar atmosférico considerando uma composição 
%   de Oxigênio (21%) e Nitrogênio (79%) apenas, a 100ºC.
%
%   t = 373.15;
%   f_mol = [0.79 0.21 0 0 0 0 0 0];
%
%   ANS: 21.8025339818354e-006
%   
%--------------------------------------------------------------------------


if  sum(frac_mol) ~= 1 %checa composição informada
    error('A soma das frações de composição é diferente de 1');
elseif frac_mol(4) ~= 0
    error('Erro: Gás Neonio não contemplado no modelo');
end


mm_el = [28.014 31.998 39.95 20.180 33.006 44.009 28.01 64.058]; %massa molar dos gases puros segundo IUPAC 2020, [g/mol]

mu = 0;
cont = 0;
vis = zeros(1, 8);
fm = zeros(1, 8);
mm = zeros(1, 8);
psi_ab = zeros(1, 8); 

coef = [0.31619*10^(-5)		0.56192*10^(-7) 	-0.24148*10^(-10)  	0.61370*10^(-14) 	250 	1500;
        0.26918*10^(-5)		0.68519*10^(-7)  	-0.29857*10^(-10) 	0.75600*10^(-14) 	250 	1500;
        0.50458*10^(-5)		0.63459*10^(-7)  	-0.17506*10^(-10) 	0.37009*10^(-14) 	250     1300;
        0                   0                   0                   0                   0       0;
        -0.41991*10^(-5) 	0.45336E-07    		-0.50749*10^(-11) 	0.15526*10^(-14) 	400 	1500;
        -0.16636*10^(-5)	0.63064*10^(-7)  	-0.26223*10^(-10) 	0.58813*10^(-14) 	250 	1500; 
        0.30012*10^(-5)		0.56504*10^(-7)  	-0.23998*10^(-10) 	0.62734*10^(-14) 	250 	1500; 
        0-.37930*10^(-5)	0.46450*10^(-7) 	-0.72760*10^(-11) 	0                   170 	1700];

    for i = 1:8, %percorre espécies
        if frac_mol(i) ~= 0  %evita o cálculo das especies com concentração nula
            cont=cont+1;
            fm(cont)= frac_mol(i);
            mm(cont)= mm_el(i);
            vis(cont)=coef(i,1)+coef(i,2)*t+coef(i,3)*t^2+coef(i,4)*t^3;
            if t<coef(i,5)
                error('A temperatura está abaixo do limite de aplicabilidade do modelo para o gas abaixo:')
            elseif t>coef(i,6)
                error('A temperatura está acima do limite de aplicabilidade do modelo para os gas abaixo:')
            end
        end
    end
    
    for a = 1:cont, %calculo psi
        for b = 1:cont,
            psi_ab(a)=psi_ab(a)+fm(b)*((1/sqrt(8))*(1+mm(a)/mm(b))^(-0.5)*(1+(vis(a)/vis(b))^(0.5)*(mm(b)/mm(a))^(0.25))^2);
        end
        mu=mu+((fm(a)*vis(a))/psi_ab(a));
    end
    y = mu;

== matlab function simulink_validacao/Recuperdor de calor CWPS/Troca de Calor/Condutividade/cond_c_ch1 ==
  data: t input; y output; frac_mol input
function y = k(t, frac_mol)
%#codegen
%
%------------------ FUNÇÃO CONDUTIVIDADE DOS GASES ------------------------
%
%   -Autor: Janderson Honório Mazzine Afonso
%   -Email: janderson.mazzine2015@engenharia.ufjf.br
%   -Ano: 2020
%
%   -Referências: 
%   [1]MATOS, M. A. A. Propriedades termofísicas de algunsgases, sólidos e  
%   da água. Aveiro: Editora da Universidade de Aveiro, 1998.
%   [2]BIRD R. B., WARREN E. S., and EDWIN N. L. Transport Phenomena. 2nd 
%   ed. New York: Jonh Wiley & Sons, 2002.
%   [3]IUPAC. Periodic Table of Elements. Disponivel em
%   <https://iupac.org/what-we-do/periodic-table-of-elements/> Acesso em
%   01 set. 2020.
%
%   -Citar como: AFONSO. Janderson H. M. Condutividade dos Gases de 
%                Combustão Aplicados em Turbinas a Gás. UFJF, 2020.
%   -Versão: 03.09.2020
%
%----------------------- DESCRIÇÃO DA FUNÇÃO ------------------------------
%
%   A presente função retorna a condutividade, em [W/m.K] de um gás puro 
%   segundo a expressão e coeficientes de regressão apresentados por Matos  
%   [1], e da mistura considerando também a correlação semiempírica 
%   desenvolvida por Wilke e apresentada no livro de Bird [2], considerando
%   as massas molares dos atomos na tabela da IUPAC [3].
%
%--------------------------- INSTRUÇÕES -----------------------------------
%
%                   [k] = cond_gas( t, frac_mol)
%
%   A temperatura de entrada deve ser dada em Kelvin [K] e as frações 
%   molares devem ser dada em um vetor com o seguinte formato:
%   
%                 (%N2 %O2 %Ar %Ne %H2O %CO2 %CO %SO2)
%
%   Caso alguma das espécies não faça parte da mistura deve ser atribuido o
%   valor 0 (zero) a sua posição no vetor. A soma das frações de cada espé-
%   cie deve ser sempre igual a 1.
%   
%   Porém, o presente modelo não contempla o gas neônio. Caso seja
%   necessário, deve-se implementar seus coeficientes na matriz.
%
%-------------------- MENSAGEM DE ERRO E AVISOS --------------------------- 
%
%   Uma mensagem de erro será exibida caso a soma das concentrações dos 
%   componentes do gás em estudo seja diferente de 1, ou caso tente-se 
%   computar um gás que possua Neônio em sua composição, o qual não é 
%   contemplado no presente modelo.
%   
%   Um aviso será exibido caso a temperatura desejada da mistura esteja
%   fora do intervalo de temperatura de algum dos gases puros que a compõe,
%   conforme a tabela abaixo:
%
%              Gas	|	T_min (K)	|	T_max (K)
%               ---------------------------------
%               N2 		  250 			  1500
%               O2		  250 			  1500
%               Ar		  110			  1300
%               Ne		  NaN			  NaN
%               H2O 	  400 			  1500
%               CO2 	  250 			  1500 
%               CO		  250 			  1500
%               SO2 	  170 			  1700
%
%---------------------------- EXEMPLOS ------------------------------------
%
%   1)Definir a condutividade do ar atmosférico considerando uma composição 
%   de Oxigênio (21%) e Nitrogênio (79%) apenas, a 100ºC.
%
%   t = 373.15;
%   f_mol = [0.79 0.21 0 0 0 0 0 0];
%   [k] = cond_gas( t, f_mol)
%
%   ANS: 30.8821778098117e-003
%   
%--------------------------------------------------------------------------


if  sum(frac_mol) ~= 1 %checa composição informada
    error('A soma das frações de composição é diferente de 1');
elseif frac_mol(4) ~= 0
    error('Erro: Gás Neonio não contemplado no modelo');
end

mm_el = [28.014 31.998 39.95 20.180 33.006 44.009 28.01 64.058]; %massa molar dos gases puros segundo IUPAC 2020, [g/mol]

k = 0;
cont = 0;
cond = zeros(1, 8);
vis = zeros(1, 8);
fm = zeros(1, 8);
mm = zeros(1, 8);
psi_ab = zeros(1, 8);


coef_cond = [0.47088*10^(-2)	0.78562*10^(-4) 	-0.26266*10^(-7) 	0.55540*10^(-11) 	250 	1500;
            0.33470*10^(-2) 	0.81930*10^(-4) 	-0.16987*10^(-7) 	0.29881*10^(-11) 	250 	1500;
            0.27132*10^(-2) 	0.55394*10^(-4) 	-0.21772*10^(-7) 	0.55268*10^(-11) 	110 	1500;
            0                   0                   0                   0                   0       0;
            -0.79293*10^(-2) 	0.76030*10^(-4) 	0.31270*10^(-7) 	-0.10805*10^(-10)	400 	1500;
            -0.95947*10^(-2) 	0.92700*10^(-4) 	-0.19366*10^(-7) 	0.32189*10^(-11) 	250 	1500;
            0.10224*10^(-2)		0.89079*10^(-4) 	-0.32557*10^(-7) 	0.89390*10^(-11) 	250 	1500;
            -0.80851*10^(-2)	0.63433*10^(-4) 	-0.13817*10^(-7) 	0.23028*10^(-11) 	300     1700];


coef_visc = [0.31619*10^(-5)	0.56192*10^(-7) 	-0.24148*10^(-10)  	0.61370*10^(-14) 	250 	1500;
            0.26918*10^(-5)		0.68519*10^(-7)  	-0.29857*10^(-10) 	0.75600*10^(-14) 	250 	1500;
            0.50458*10^(-5)		0.63459*10^(-7)  	-0.17506*10^(-10) 	0.37009*10^(-14) 	250     1300;
            0                   0                   0                   0                   0       0;
            -0.41991*10^(-5) 	0.45336E-07    		-0.50749*10^(-11) 	0.15526*10^(-14) 	400 	1500;
            -0.16636*10^(-5)	0.63064*10^(-7)  	-0.26223*10^(-10) 	0.58813*10^(-14) 	250 	1500; 
            0.30012*10^(-5)		0.56504*10^(-7)  	-0.23998*10^(-10) 	0.62734*10^(-14) 	250 	1500; 
            0-.37930*10^(-5)	0.46450*10^(-7) 	-0.72760*10^(-11) 	0                   170 	1700];

    for i = 1:8, %percorre espécies
        if frac_mol(i) ~= 0  %evita o cálculo das especies com concentração nula
            cont=cont+1;
            fm(cont)= frac_mol(i);
            mm(cont)= mm_el(i);
            vis(cont)=coef_visc(i,1)+coef_visc(i,2)*t+coef_visc(i,3)*t^2+coef_visc(i,4)*t^3;
            cond(cont)=coef_cond(i,1)+coef_cond(i,2)*t+coef_cond(i,3)*t^2+coef_cond(i,4)*t^3;
            if t<coef_visc(i,5)||t<coef_cond(i,5)
                error('A temperatura está abaixo do limite de aplicabilidade do modelo para o gas abaixo:')
                %disp(n_esp(i));
            elseif t>coef_visc(i,6)||t>coef_cond(i,6)
                error('A temperatura está acima do limite de aplicabilidade do modelo para os gas abaixo:')
                %disp(n_esp(i));
            end
        end
    end
    
    for a = 1:cont, %calculo psi
        for b = 1:cont,
            psi_ab(a)=psi_ab(a)+fm(b)*((1/sqrt(8))*(1+mm(a)/mm(b))^(-0.5)*(1+(vis(a)/vis(b))^(0.5)*(mm(b)/mm(a))^(0.25))^2);
        end
        k=k+((fm(a)*cond(a))/psi_ab(a));
    end    
y = k;

== matlab function simulink_validacao/Recuperdor de calor CWPS/Troca de Calor/Cp Cr e Cmin/cp_c_ch ==
  data: t input; y output; frac_mol input
function y = cp(t,frac_mol)
%#codegen
%
%----------------- FUNÇÃO CALOR ESPECÍFICO DOS GASES ----------------------
%
%   -Autor: Janderson Honório Mazzine Afonso
%   -Email: janderson.mazzine2015@engenharia.ufjf.br
%   -Ano: 2020
%   -Referência: BUCKER, D.; SPAN, R.; WAGNER, W. Thermodynamic property 
%                models for moist air and combustion gases. J. Eng. Gas 
%                Turbines Power, v. 125, n. 1, p. 374-384, 2003.
%                https://doi.org/10.1115/1.1520154
%   -Citar como: AFONSO. Janderson H. M. Propriedade dos Gases de Combustão
%                Aplicados em Turbinas a Gás - Calor específico. UFJF,
%                2020.
%   -Versão: 14.05.2020
%
%----------------------- DESCRIÇÃO DA FUNÇÃO ------------------------------
%
%   A presente função retorna o calor específico a pressão constante em  
%   J/kg.K de uma mistura de gases que compõe o ar e produtos da combustão
%   para temperaturas entre 200 e 3300 Kelvin de acordo com o modelo pro- 
%   posto por BUCKER, SPAN e WAGNER (2003) em seu trabalho "Thermodynamic 
%   Property Model for Moist Air and Combustion Gases" a partir da tempe-
%   ratura da mistura e sua composição molar.
%
%--------------------------- INSTRUÇÕES -----------------------------------
%
%                       [cp] = cp( t, frac_mol)
%
%   A temperatura de entrada deve ser dada em Kelvin [K], e a composição 
%   molar da mistura e a base dimensional de cálculo. As frações molares 
%   devem ser dada em um vetor com o seguinte formato:
%
%                 (%N2 %O2 %Ar %Ne %H2O %CO2 %CO %SO2)
%
%   Caso alguma das espécies não faça parte da mistura deve ser atribuido o
%   valor 0 (zero) a sua posição no vetor. A soma das frações de cada espé-
%   cie deve ser sempre igual a 1.
%
%------------------------ MENSAGEM DE ERRO -------------------------------- 
%
%   Uma mensagem de erro será exibida caso a temperatura
%   informada esteja fora dos limites de validade do modelo (entre 200 e
%   3300 K) ou caso a soma das concentrações dos componentes do gás em
%   estudo seja diferente de 1.
%
%---------------------------- EXEMPLOS ------------------------------------
%
%   1)Definir o calor específico a pressão constante do ar atmosférico
%   considerando uma composição de Oxigênio (21%) e Nitrogênio (79%)   
%   apenas, a 30ºC.
%
%   t = 303.15;
%   f_mol = [0.79 0.21 0 0 0 0 0 0]
%   [cp] = cp( t, f_mol )
%
%   ANS:
%   cp = 1.01438564661116e+003
%
%--------------------------------------------------------------------------


if t < 200 || t > 3300 %checa aplicabilidade do modelo
    error('Temperatura informada fora do intervalo de validade do modelo(200 K < T < 3300 K)')
elseif sum(frac_mol) ~= 1 %checa composição informada
    error('A soma das frações de composição é diferente de 1')
end

b_i = [0.00 -1.50 -1.25 -0.75 -0.50 -0.25 0.25 0.50 0.75 1.00];
%b_i : vetor de coeficientes bi
   
a_ki = [2.475830346*10^6 -2.815239891*10^4 1.116401165*10^5 -8.147644187*10^5 2.185120405*10^6 -2.978031305*10^6 -1.308008001*10^6 4.305948510*10^5 -8.082302563*10^4 6.622545214*10^3;
        6.408242565*10^5 -1.599937045*10^3 9.984801256*10^3 -1.280873444*10^5 4.186599156*10^5 -6.720142804*10^5 -3.799977202*10^5 1.378691801*10^5 -2.806954185*10^4 2.459943097*10^3;
        2.078618000*10^1 0 0 0 0 0 0 0 0 0; 
        2.078618000*10^1 0 0 0 0 0 0 0 0 0;
        -4.747782033*10^6 4.799919289*10^4 -1.931588954*10^5 1.460728340*10^6 -4.000075762*10^6 5.576209858*10^6 2.570488297*10^6 -8.670521019*10^5 1.666429390*10^5 -1.396634620*10^4;
        1.103695150*10^6 -1.365096910*10^4 5.357704944*10^4 -3.816063864*10^5 1.008950325*10^6 -1.352938737*10^6 -5.701809626*10^5 1.828513133*10^5 -3.329618224*10^4 2.635366727*10^3;
        2.670755728*10^6 -2.715629936*10^4 1.096509012*10^5 -8.303525865*10^5 2.269213594*10^6 -3.151865706*10^6 -1.438126165*10^6 4.824833432*10^5 -9.227524508*10^4 7.701550175*10^3;
        -2.076653674*10^6 2.589571253*10^4 -1.012523438*10^5 7.161863952*10^5 -1.889754780*10^6 2.535020356*10^6 1.082842148*10^6 -3.524395911*10^5 6.552035769*10^4 -5.325634796*10^3;]; 
%a_ki : matriz coef. ak_i, i = (1:10) (colunas) e especies (linhas)

t_0 = 273.15; %Temperatura de referência, em K
cp = 0;
      
mm_esp = [28.014 31.998 39.948 20.180 18.015 40.019 28.009 64.063]; 
%mm_esp : massa molar das espécies
for i = 1:8, %Percorre espécies
  cp_esp = 0;
  if frac_mol(i) > 0  %evita o cálculo das especies com concentração nula
      for j = 1:10, %percorre coeficientes
          cp_esp = cp_esp + a_ki(i,j)*((t/t_0)^b_i(j));
      end
  end
  cp = cp + cp_esp*frac_mol(i)*(1000/mm_esp(i));
end
 
y = cp;
